simulink model "SensorFusion_Controller_Model"  (R2025a)
settings: Solver=VariableStepAuto  StartTime=0.0  StopTime=inf  FixedStep=1  RelTol=1e-3
undefined symbols (not defined in the file): DiscIntNeverNeededParam
libraries: simulink x17
(part 4 of 4)

== stateflow chart SensorFusion_Controller_Model/Rule Based Flood Controller_1/Water Pump and Sluice Gate Controller ==
  state AUTO_MODE
    entry:
    controlMode=0;
    state NORMAL
      entry:
      PumpCmd=0;
      GateCmd=0;
      Auto_SirenCmd=false;
    state AI_EARLY_MITIGATION
      entry:
      AI_EarlyMitigationActive=1;
      during:
      controlMode = 0;
      PumpCmd = 0;
      GateCmd = 0;
      Auto_SirenCmd = false;
      if Rainfall_Norm >= 0.8 && RiverLevel_Norm >= 0.8
      PumpCmd = 1;
      GateCmd = 1;
      elseif Rainfall_Norm >= RiverLevel_Norm
      PumpCmd = 1;
      else
      GateCmd = 1;
      end
      exit:
      AI_EarlyMitigationActive=0;
    state ALERT
      during:
      PumpCmd = 0;
      GateCmd = 0;
      Auto_SirenCmd = false;
      if Flood_Type == 1
      GateCmd = 1;      % 30%
      elseif Flood_Type == 2
      PumpCmd = 1;      % 30%
      elseif Flood_Type == 3
      PumpCmd = 1;      % 30%
      GateCmd = 1;      % 30%
      end
    state WARNING
      during:
      PumpCmd = 0;
      GateCmd = 0;
      Auto_SirenCmd = false;
      if Flood_Type == 1
      GateCmd = 2;      % 70%
      elseif Flood_Type == 2
      PumpCmd = 2;      % 70%
      elseif Flood_Type == 3
      PumpCmd = 2;      % 70%
      GateCmd = 2;      % 70%
      end
    state DANGER
      entry:
      PumpCmd = 3;          % 100%
      GateCmd = 3;          % 100%
      Auto_SirenCmd = true;
    (default) -> NORMAL
    AI_EARLY_MITIGATION -> NORMAL [order 1] : [AI_FloodFlag == 0 || Confidence <= 0.3]
    NORMAL -> AI_EARLY_MITIGATION [order 2] : [FRI < 0.3 && AI_FloodFlag==1&&Confidence>0.61]
    ALERT -> NORMAL [order 2] : [FRI < 0.29]
    NORMAL -> ALERT [order 1] : [FRI >= 0.3]
    AI_EARLY_MITIGATION -> ALERT [order 2] : [FRI >= 0.3]
    WARNING -> ALERT [order 2] : [FRI < 0.56]
    ALERT -> WARNING [order 1] : [FRI >= 0.6]
    DANGER -> WARNING : [FRI <= 0.76]
    WARNING -> DANGER [order 1] : [FRI >= 0.8]
  state MANUAL_MODE
    state MANUAL_MODE
      during:
      controlMode = 1;
      PumpCmd = Manual_PumpLevel;
      GateCmd = Manual_GateLevel;
      if Manual_PumpLevel > 3
      PumpCmd = 0;
      else
      PumpCmd = Manual_PumpLevel;
      end
      if Manual_GateLevel > 3
      GateCmd = 0;
      else
      GateCmd = Manual_GateLevel;
      end
    (default) -> MANUAL_MODE.MANUAL_MODE
  (default) -> AUTO_MODE
  AUTO_MODE -> MANUAL_MODE : [Manual_Enable==1]
  MANUAL_MODE -> AUTO_MODE : [Manual_Enable==0]
  data: FRI input; Flood_Type input; PumpCmd output; GateCmd output; Auto_SirenCmd output; Manual_Enable input; controlMode output; Manual_GateLevel input; Manual_PumpLevel input; AI_FloodFlag input; Confidence input; AI_EarlyMitigationActive output; Rainfall_Norm input; RiverLevel_Norm input

== matlab function SensorFusion_Controller_Model/Sensor Fusion/MATLAB Function11 ==
  data: noisy_input input; x_est output
function x_est = kalmanFilter(noisy_input)

persistent x P
if isempty(x), x = noisy_input; end
if isempty(P), P = 1; end


Q = 1e-4;   % process noise covariance
R = 1e-3;   % measurement noise covariance
% R > Q : filter trusts its own prediction slightly more than noise
% measurement

% prediction
x_pred = x;
P_pred = P + Q;

% update
K = P_pred / (P_pred + R);
x = x_pred + K*(noisy_input - x_pred);
P = (1 - K)*P_pred;

x_est = max(0, x);

== matlab function SensorFusion_Controller_Model/Sensor Fusion/MATLAB Function3 ==
  data: noisy_input input; x_est output
function x_est = kalmanFilter(noisy_input)

persistent x P
if isempty(x), x = noisy_input; end
if isempty(P), P = 1; end


Q = 1e-4;   % process noise covariance
R = 1e-3;   % measurement noise covariance
% R > Q : filter trusts its own prediction slightly more than noise
% measurement

% prediction
x_pred = x;
P_pred = P + Q;

% update
K = P_pred / (P_pred + R);
x = x_pred + K*(noisy_input - x_pred);
P = (1 - K)*P_pred;

x_est = max(0, x);
